simulink model "doc_hammingcode"  (R2014a)
settings: Solver=ode45  SolverMode=SingleTasking  StartTime=0.0  StopTime=inf  RelTol=1e-3
undefined symbols (not defined in the file or in its folder): gfprimfd
libraries: commblkcod2 x2, commrandsrc2 x1, commchan3 x1, commsink2 x1, simulink x1
settings Model: Creator=The MathWorks Inc.
settings DataIOCC: SignalLoggingSaveFormat=ModelDataLogs  SaveOutput=off  SaveTime=off  SignalLoggingName=sigsOut
settings OptimizationCC: BooleanDataType=off  InlineParams=on  ExpressionDepthLimit=2147483647
settings DebuggingCC: AlgebraicLoopMsg=error  SaveWithParameterizedLinksMsg=none  UnderspecifiedInitializationDetection=Classic  SignalResolutionControl=TryResolveAllWithWarning  SolverPrmCheckMsg=none  MultiTaskDSMMsg=warning  MultiTaskCondExecSysMsg=none  FcnCallInpInsideContextMsg=UseLocalSettings  StateNameClashWarn=warning  StrictBusMsg=None
settings HardwareCC: TargetUnknown=on
settings RTWCC: IncludeERTFirstTime=on
settings GRTTargetCC: CombineOutputUpdateFcns=off  GRTInterface=on

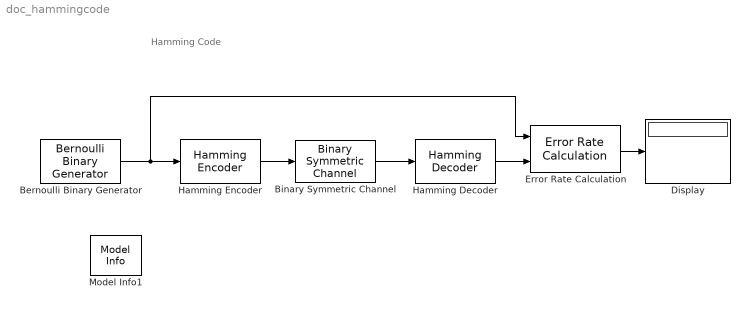
== system doc_hammingcode ==
  note: Hamming Code
  Bernoulli Binary Generator : commrandsrc2/Bernoulli Binary Generator  P=0.5  seed=61  Ts=1  frameBased=on  sampPerFrame=4  orient=off  outDataType=double
  Binary Symmetric Channel : commchan3/Binary Symmetric Channel  P=0.01  s=2137  E=off  outDtype=double
  Display : Display
  Error Rate Calculation : commsink2/Error Rate Calculation  N=0  st_delay=0  cp_mode=Entire frame  subframe=[]  PMode=Port  WsName=ErrorVec  RsMode2=off  stop=on  numErr=100  maxBits=1e6
  Hamming Decoder : commblkcod2/Hamming Decoder  n=7  k=gfprimfd(3,'min')
  Hamming Encoder : commblkcod2/Hamming Encoder  n=7  k=gfprimfd(3,'min')
  Model Info1 : simulink/Model-Wide Utilities/Model Info  InitialBlockCM=None  BlockCM=None  Frame=on  DisplayStringWithTags=Info  HorizontalTextAlignment=Center  LeftAlignmentValue=0.5  SourceBlockDiagram=doc_hammingcode  TagMaxNumber=20
  wires:
  Error Rate Calculation/1 -> Display/1
  Bernoulli Binary Generator/1 -> Hamming Encoder/1, Error Rate Calculation/1
  Hamming Decoder/1 -> Error Rate Calculation/2
  Hamming Encoder/1 -> Binary Symmetric Channel/1
  Binary Symmetric Channel/1 -> Hamming Decoder/1
